simulink model "pendulum"  (R2020a)
settings: Solver=FixedStepAuto  StartTime=0.0  StopTime=t_stop  FixedStep=.01  RelTol=1e-3
values from neighbouring files (symbols this model uses):
  c = 5    [main_doublependulum.m]    (also in main_pendulum.m = 0.8; main_pendulum_arch.m; pendulum_simulation.m = 0.4)
  g = 9.8    [main_doublependulum.m]    (also in main_pendulum.m; main_pendulum_arch.m; pendulum_simulation.m)
  Io = m*l^2    (= 2.5)    [main_pendulum.m]    (also in pendulum_simulation.m = 0.18)
  l = 42*(1/100)    (= 0.42)    [main_doublependulum.m]    (also in main_pendulum.m = 0.5; main_pendulum_arch.m; pendulum_simulation.m = 0.3)
  m = 2    [main_doublependulum.m]    (also in main_pendulum.m = 10; main_pendulum_arch.m; pendulum_simulation.m)
  u10 = 50*pi/180    (= 0.872664625997)    [main_pendulum.m]    (also in pendulum_simulation.m)
settings Model: Creator=thill  LastModifiedBy=thill

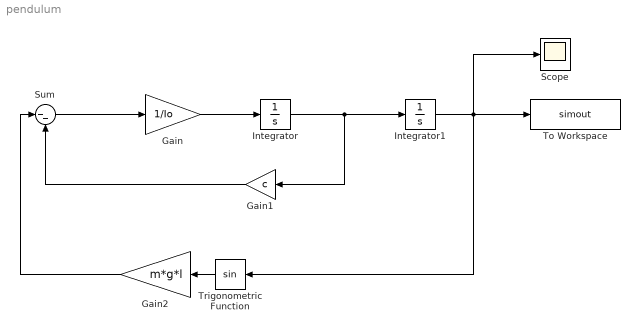
== system pendulum ==
  Gain : Gain  Gain=1/Io
  Gain1 : Gain  Gain=c
  Gain2 : Gain  Gain=m*g*l
  Integrator : Integrator
  Integrator1 : Integrator  InitialCondition=u10
  Scope : Scope
  Sum : Sum  Inputs=|--
  To Workspace : ToWorkspace  VariableName=simout  SaveFormat=Timeseries  SampleTime=-1
  Trigonometric Function : Trigonometry  OutputSignalType=real
  wires:
  Sum/1 -> Gain/1
  Gain/1 -> Integrator/1
  Integrator/1 -> Integrator1/1, Gain1/1
  Integrator1/1 -> Trigonometric Function/1, Scope/1, To Workspace/1
  Gain1/1 -> Sum/2
  Trigonometric Function/1 -> Gain2/1
  Gain2/1 -> Sum/1
